simulink model "Controller_PP_testV1"  (R2021a)
settings: Solver=FixedStepDiscrete  StartTime=0.0  StopTime=inf  FixedStep=0.05  RelTol=1e-3
PostLoadFcn:
  | , if any(exist('dsrtsu_mdlpostloadfcn', 'file') == [2, 3, 6]), try dsrtsu_mdlpostloadfcn('Execute', bdroot); catch fprintf('Error in PostLoadFcn (dsrtsu_mdlpostloadfcn) for model "%s":\n %s\n', bdroot, lasterr); end, end,
model workspace (MAT data in the model file):
  DLC_kr = [-5.84862481044e-05 -6.43095507895e-05 -7.01328534794e-05 -7.5956156174e-05 -8.17794588731e-05 -8.76027615758e-05 -9.34260642811e-05 -9.92493669872e-05 -0.000105072669692 -0.000110895972393 -0.000116719275087 -0.000122542545808 ... (2080 elements, 1x2080)]
  DLC_thetar = [1.57172954906 1.57172588114 1.57172186534 1.57171750165 1.57171279008 1.57170773062 1.57170232328 1.57169656806 1.57169046495 1.57168401395 1.57167721507 1.57167006831 ... (2080 elements, 1x2080)]
  DLC_xr = [-0.00056695162723 -0.000622594591628 -0.000678008043004 -0.000733171198692 -0.000788063276025 -0.000842663492338 -0.000896951064963 -0.000950905211235 -0.00100450514849 -0.00105773009405 -0.00111055926527 -0.00116297187948 ... (2080 elements, 1x2080)]
  DLC_yr = [0.59999973213 0.659739817002 0.719479902091 0.779219987412 0.838960072984 0.898700158824 0.958440244948 1.01818033138 1.07792041812 1.1376605052 1.19740059264 1.25714068045 ... (2080 elements, 1x2080)]
  Fliter_ = 0.5
  Fliter_k = 1
  Iz = 1650
  SL_ROS_VariableLengthArrays_MaxSizes : object (value not decoded)
  a = 1
  b = 1.8
  cf = -120000
  cr = -120000
  factor_str = 0.15
  k1 = [0.258198889801 0.258198889749 0.258198889743 0.258198889805 0.258198889772 0.258198889764 0.258198889767 0.258198889768 0.258198889748 0.258198889747 0.258198889747 0.258198889747 ... (1000 elements, 1x1000)]
  k2 = [0.000225641086743 0.000451280556994 0.000676916794375 0.000902548182649 0.00112817310577 0.00135378994806 0.00157939709421 0.00180499292937 0.00203057583924 0.00225614421016 0.00248169642913 0.00270723088396 ... (1000 elements, 1x1000)]
  k3 = [1.8072435186 1.8072437178 1.80724404966 1.8072445143 1.80724511184 1.80724584231 1.80724670582 1.80724770248 1.80724883243 1.8072500958 1.80725149277 1.80725302351 ... (1000 elements, 1x1000)]
  k4 = [0.000229144738699 0.000458288056581 0.000687428532897 0.000916564747031 0.00114569527856 0.00137481870732 0.00160393361347 0.00183303857755 0.00206213218056 0.00229121300401 0.00252027963002 0.00274933064131 ... (1000 elements, 1x1000)]
  kr = [3.43040952456 5.20354947673 6.57526776383 5.89663744443 5.05963864905 4.19207203133 3.37422700169 2.64183787985 2.00068698258 1.44046440991 0.943931458435 0.491794250204 ... (89883 elements, 89883x1)]
  m = 1500
  straight_kr = [0 0 0 0 0 0 0 0 0 0 0 0 ... (10000 elements, 10000x1)]
  straight_thetar = [1.5708 1.5708 1.5708 1.5708 1.5708 1.5708 1.5708 1.5708 1.5708 1.5708 1.5708 1.5708 ... (10000 elements, 10000x1)]
  straight_xr = [0 0 0 0 0 0 0 0 0 0 0 0 ... (10000 elements, 10000x1)]
  straight_yr = [0.01 0.02 0.03 0.04 0.05 0.06 0.07 0.08 0.09 0.1 0.11 0.12 ... (10000 elements, 10000x1)]
  thetar = [0.0108871889919 0.137918447215 0.259619297152 0.371627288769 0.47112102891 0.556859678388 0.628810120477 0.687658443901 0.734398145371 0.77005371967 0.795522448239 0.811495552059 ... (89883 elements, 89883x1)]
  xr = [399944.786619 399944.805491 399944.823621 399944.841077 399944.857922 399944.874223 399944.890046 399944.905456 399944.920519 399944.935301 399944.949866 399944.964282 ... (89883 elements, 89883x1)]
  xr_init = 3407363.99438
  yr = [3406937.32043 3406937.32184 3406937.3255 3406937.33122 3406937.33879 3406937.34802 3406937.35871 3406937.37066 3406937.38366 3406937.39752 3406937.41203 3406937.427 ... (89883 elements, 89883x1)]
  yr_init = 400335.964759
undefined symbols (not defined in the file or in its folder): Data, Data_SL_Info
libraries: robotlib x5, simulink_extras x3
(part 2 of 2)

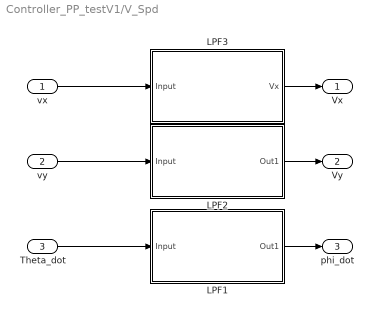
== system Controller_PP_testV1/V_Spd ==
  vx : Inport
  vy : Inport  Port=2
  Theta_dot : Inport  Port=3
  LPF1 : Subsystem  TreatAsAtomicUnit=on
  LPF2 : Subsystem  TreatAsAtomicUnit=on
  LPF3 : Subsystem  TreatAsAtomicUnit=on
  Vx : Outport  VectorParamsAs1DForOutWhenUnconnected=off
  Vy : Outport  Port=2  VectorParamsAs1DForOutWhenUnconnected=off
  phi_dot : Outport  Port=3  VectorParamsAs1DForOutWhenUnconnected=off
  wires:
  Theta_dot/1 -> LPF1/1(Input)
  LPF1/1(Out1) -> phi_dot/1
  LPF2/1(Out1) -> Vy/1
  LPF3/1(Vx) -> Vx/1
  vx/1 -> LPF3/1(Input)
  vy/1 -> LPF2/1(Input)

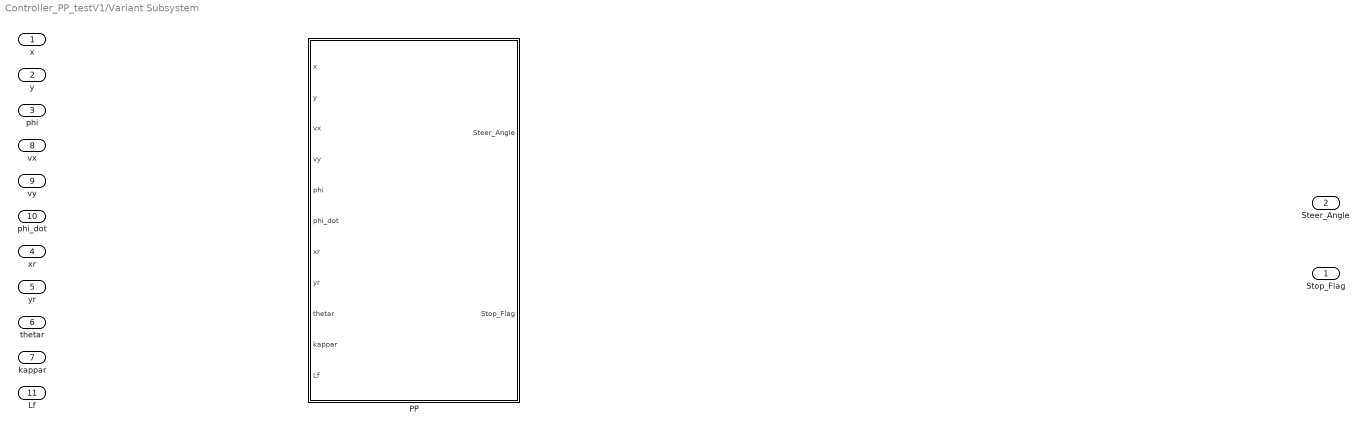
== system Controller_PP_testV1/Variant Subsystem ==
  x : Inport
  y : Inport  Port=2
  phi : Inport  Port=3
  xr : Inport  Port=4
  yr : Inport  Port=5
  thetar : Inport  Port=6
  kappar : Inport  Port=7
  vx : Inport  Port=8
  vy : Inport  Port=9
  phi_dot : Inport  Port=10
  Lf : Inport  Port=11
  PP : Subsystem  VariantControl=Controller == 5
  Stop_Flag : Outport  VectorParamsAs1DForOutWhenUnconnected=off
  Steer_Angle : Outport  Port=2  VectorParamsAs1DForOutWhenUnconnected=off

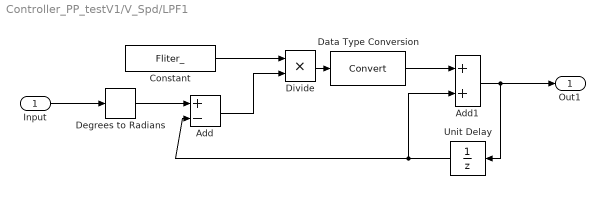
== system Controller_PP_testV1/V_Spd/LPF1 ==
  Input : Inport
  Add : Sum  Inputs=+-
  Add1 : Sum
  Constant : Constant  Value=Fliter_
  Data Type Conversion : DataTypeConversion
  Degrees to Radians : simulink_extras/Transformations/Degrees to Radians
  Divide : Product  Inputs=**
  Unit Delay : UnitDelay  SampleTime=-1  HasFrameUpgradeWarning=on
  Out1 : Outport  VectorParamsAs1DForOutWhenUnconnected=off
  wires:
  Divide/1 -> Data Type Conversion/1
  Input/1 -> Degrees to Radians/1
  Constant/1 -> Divide/1
  Add/1 -> Divide/2
  Data Type Conversion/1 -> Add1/1
  Add1/1 -> Unit Delay/1, Out1/1
  Unit Delay/1 -> Add/2, Add1/2
  Degrees to Radians/1 -> Add/1

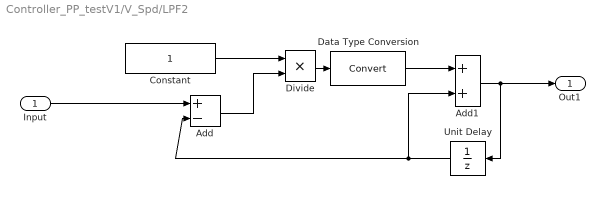
== system Controller_PP_testV1/V_Spd/LPF2 ==
  Input : Inport
  Add : Sum  Inputs=+-
  Add1 : Sum
  Constant : Constant
  Data Type Conversion : DataTypeConversion
  Divide : Product  Inputs=**
  Unit Delay : UnitDelay  SampleTime=-1  HasFrameUpgradeWarning=on
  Out1 : Outport  VectorParamsAs1DForOutWhenUnconnected=off
  wires:
  Divide/1 -> Data Type Conversion/1
  Constant/1 -> Divide/1
  Add/1 -> Divide/2
  Data Type Conversion/1 -> Add1/1
  Add1/1 -> Unit Delay/1, Out1/1
  Unit Delay/1 -> Add/2, Add1/2
  Input/1 -> Add/1

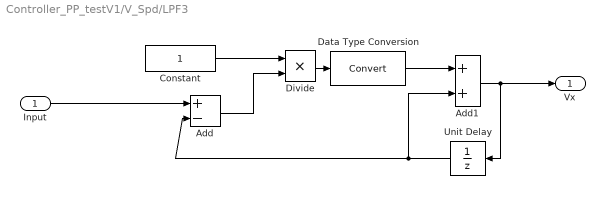
== system Controller_PP_testV1/V_Spd/LPF3 ==
  Input : Inport
  Add : Sum  Inputs=+-
  Add1 : Sum
  Constant : Constant
  Data Type Conversion : DataTypeConversion
  Divide : Product  Inputs=**
  Unit Delay : UnitDelay  SampleTime=-1  HasFrameUpgradeWarning=on
  Vx : Outport  VectorParamsAs1DForOutWhenUnconnected=off
  wires:
  Input/1 -> Add/1
  Unit Delay/1 -> Add1/2, Add/2
  Add1/1 -> Vx/1, Unit Delay/1
  Data Type Conversion/1 -> Add1/1
  Add/1 -> Divide/2
  Constant/1 -> Divide/1
  Divide/1 -> Data Type Conversion/1

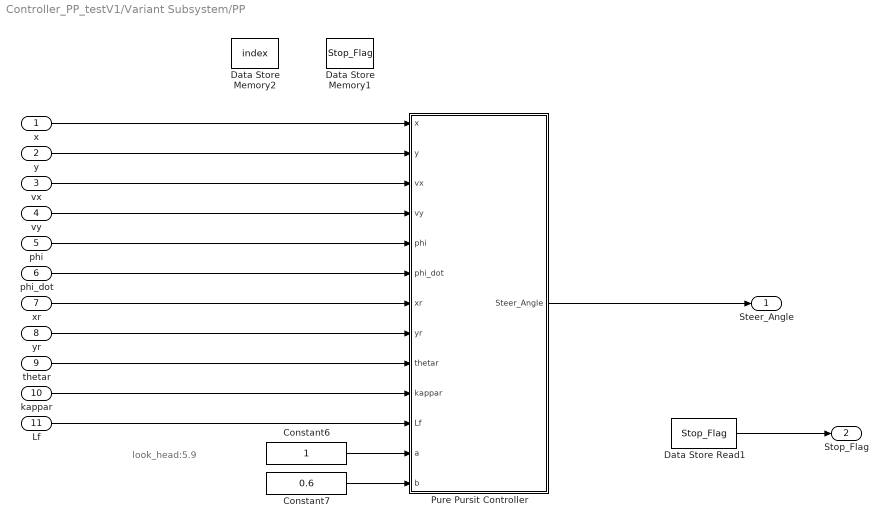
== system Controller_PP_testV1/Variant Subsystem/PP ==
  note: look_head:5.9
  x : Inport
  y : Inport  Port=2
  vx : Inport  Port=3
  vy : Inport  Port=4
  phi : Inport  Port=5
  phi_dot : Inport  Port=6
  xr : Inport  Port=7
  yr : Inport  Port=8
  thetar : Inport  Port=9
  kappar : Inport  Port=10
  Lf : Inport  Port=11
  Constant6 : Constant
  Constant7 : Constant  Value=0.6
  Data Store Memory1 : DataStoreMemory  DataStoreName=Stop_Flag  ReadBeforeWriteMsg=warning  WriteAfterWriteMsg=warning  WriteAfterReadMsg=warning  ShowAdditionalParam=off  OutDataTypeStr=double
  Data Store Memory2 : DataStoreMemory  DataStoreName=index  ReadBeforeWriteMsg=warning  WriteAfterWriteMsg=warning  WriteAfterReadMsg=warning  ShowAdditionalParam=off  OutDataTypeStr=double
  Data Store Read1 : DataStoreRead  DataStoreName=Stop_Flag  IndexOptions=Index vector (dialog)  Indices=1  OutputSizes=1
  Pure Pursit Controller : MATLAB Function  TreatAsAtomicUnit=on
  Steer_Angle : Outport
  Stop_Flag : Outport  Port=2
  wires:
  phi_dot/1 -> Pure Pursit Controller/6(phi_dot)
  Constant7/1 -> Pure Pursit Controller/13(b)
  vx/1 -> Pure Pursit Controller/3(vx)
  y/1 -> Pure Pursit Controller/2(y)
  thetar/1 -> Pure Pursit Controller/9(thetar)
  xr/1 -> Pure Pursit Controller/7(xr)
  Constant6/1 -> Pure Pursit Controller/12(a)
  vy/1 -> Pure Pursit Controller/4(vy)
  yr/1 -> Pure Pursit Controller/8(yr)
  x/1 -> Pure Pursit Controller/1(x)
  kappar/1 -> Pure Pursit Controller/10(kappar)
  Pure Pursit Controller/1(Steer_Angle) -> Steer_Angle/1
  phi/1 -> Pure Pursit Controller/5(phi)
  Data Store Read1/1 -> Stop_Flag/1
  Lf/1 -> Pure Pursit Controller/11(Lf)

== matlab function Controller_PP_testV1/MATLAB Function ==
  data: u input; xr output; yr output
function [xr,yr] = fcn(u)
xr = u(:,1);
yr = u(:,2);
end

== matlab function Controller_PP_testV1/MATLAB Function1 ==
  data: x input; y input; cones_real_heading input; cones_real_center_x input; cones_real_center_y input; new_pose data_store_memory

function fcn(x,y,cones_real_heading,cones_real_center_x,cones_real_center_y)
coder.extrinsic('plot');
%coder.extrinsic('equal');
star_pose_x = 0;   %先验8字绕环车辆起始x位置 m
star_pose_y = -2.5;%先验8字绕环车辆起始y位置 m
r = 9.125;         %先验8字绕环圆的半径
lane_width = 3;    %先验8字绕环车道宽 m
% cones_interval = 5;%先验8字绕环纵向锥桶间距 m
persistent flag  
if isempty(flag)
    flag = 0;
end
global new_pose
%% 建立先验8字路径
if flag == 0
    refPoses = zeros(191,2);
    cones_origin_poses = zeros(4,2);
    index =1;
    refPoses(1,:)=[star_pose_x,star_pose_y];
    for i =1:10
        refPoses(index+i,:)=[star_pose_x,star_pose_y+1.3*i];
    end
    index = index+20;
    for i=1:20
         refPoses(index+i,:)=[star_pose_x+r-r*cos(i*(pi/20)),r*sin(i*(pi/20))+15+star_pose_y];
    end
    index=index+20;
    for i=1:20
         refPoses(index+i,:)=[star_pose_x+r-r*cos(pi+i*(pi/20)),r*sin(pi+i*(pi/20))+15+star_pose_y];
    end
    index=index+20;
    for i=1:20
         refPoses(index+i,:)=[star_pose_x+r-r*cos(i*(pi/20)),r*sin(i*(pi/20))+15+star_pose_y];
    end
    index=index+20;
    for i=1:20
         refPoses(index+i,:)=[star_pose_x+r-r*cos(pi+i*(pi/20)),r*sin(pi+i*(pi/20))+15+star_pose_y];
    end
    index=index+20;
    for i=1:20
        refPoses(index+i,:)=[star_pose_x-r+r*cos(i*(pi/20)),r*sin(i*(pi/20))+15+star_pose_y];
    end
    index=index+20;
    for i=1:20
        refPoses(index+i,:)=[star_pose_x-r+r*cos(pi+i*(pi/20)),r*sin(pi+i*(pi/20))+15+star_pose_y];
    end
    index=index+20;
    for i=1:20
        refPoses(index+i,:)=[star_pose_x-r+r*cos(i*(pi/20)),r*sin(i*(pi/20))+15+star_pose_y];
    end
    index=index+20;
    for i=1:20
        refPoses(index+i,:)=[star_pose_x-r+r*cos(pi+i*(pi/20)),r*sin(pi+i*(pi/20))+15+star_pose_y];
    end
    index=index+20;
    for i =1:10
        refPoses(index+i,:)=[star_pose_x,star_pose_y+17+1.3*i];
    end
%     index =1;
%     refPoses(1,:)=[star_pose_x,star_pose_y];
%     for i =1:5
%         refPoses(index+i,:)=[star_pose_x,star_pose_y+2.6*i];
%     end
%     index = index+5;
%     for i=1:10
%          refPoses(index+i,:)=[star_pose_x+r-r*cos(i*(pi/10)),r*sin(i*(pi/10))+15+star_pose_y];
%     end
%     index=index+10;
%     for i=1:10
%          refPoses(index+i,:)=[star_pose_x+r-r*cos(pi+i*(pi/10)),r*sin(pi+i*(pi/10))+15+star_pose_y];
%     end
%     index=index+10;
%     for i=1:10
%          refPoses(index+i,:)=[star_pose_x+r-r*cos(i*(pi/10)),r*sin(i*(pi/10))+15+star_pose_y];
%     end
%     index=index+10;
%     for i=1:10
%          refPoses(index+i,:)=[star_pose_x+r-r*cos(pi+i*(pi/10)),r*sin(pi+i*(pi/10))+15+star_pose_y];
%     end
%     index=index+10;
%     for i=1:10
%         refPoses(index+i,:)=[star_pose_x-r+r*cos(i*(pi/10)),r*sin(i*(pi/10))+15+star_pose_y];
%     end
%     index=index+10;
%     for i=1:10
%         refPoses(index+i,:)=[star_pose_x-r+r*cos(pi+i*(pi/10)),r*sin(pi+i*(pi/10))+15+star_pose_y];
%     end
%     index=index+10;
%     for i =1:5
%         refPoses(index+i,:)=[star_pose_x,star_pose_y+17+2.6*i];
%     end
    %figure(1);
    %% 建立先验初始4个黄色锥桶位置
    cones_poses = [star_pose_x-lane_width/2,star_pose_y; %根据赛道初始位置确定4个锥桶位置。
                   star_pose_x+lane_width/2,star_pose_y;
                   star_pose_x-lane_width/2,star_pose_y+5;
                   star_pose_x+lane_width/2,star_pose_y+5;];
    
%    plot(cones_poses(:,1),cones_poses(:,2),'ro'); %画锥桶
 %   axis equal;
 %   hold on;
  %   plot(refPoses(:,1),refPoses(:,2),'bo');%画路径
    %% 建立假设实际4个黄色锥桶的位置
    %模拟4个锥桶位置，通过平移旋转先验锥桶位置，并且添加随机数模拟实际摆放误差。
    %先求出4个黄色锥桶的重心位置
    cones_center_origin_x =sum(cones_poses(:,1))/4;
    cones_center_origin_y =sum(cones_poses(:,2))/4;
%   plot(cones_center_origin_x,cones_center_origin_y,'*');
    %确定当前4个锥桶的方位角(航向角)
    cones_origin_heading = atan2d(refPoses(2,2) -refPoses(1,2) ,refPoses(2,1) -refPoses(1,1));
    diff_cones_heading =-(cones_real_heading - cones_origin_heading);
    %先将锥桶重心平移到原点
    cones_origin_poses(:,1) = cones_poses(:,1) - cones_center_origin_x;
    cones_origin_poses(:,2) = cones_poses (:,2)- cones_center_origin_y;
    %旋转
    eul = [deg2rad(diff_cones_heading) 0 0];
    rotation_matrix_ = eul2rotm(eul);
    rotation_matrix_ = rotation_matrix_(1:2,:);
    cones_poses_real = cones_origin_poses * rotation_matrix_;
    %从重心平移回先验锥桶重心
    cones_poses_real(:,1) = cones_poses_real(:,1) + cones_center_origin_x;
    cones_poses_real(:,2) = cones_poses_real(:,2) + cones_center_origin_y;
    %平移到期望预设锥桶位置
    cones_poses_real(:,1) = cones_poses_real(:,1) + (cones_real_center_x -cones_center_origin_x);
    cones_poses_real(:,2) = cones_poses_real(:,2) + (cones_real_center_y -cones_center_origin_y);
    %加上随机数，模拟锥桶摆放
    cones_poses_real(1,:) = cones_poses_real(1,:);
    cones_poses_real(2,:) = cones_poses_real(2,:);
    cones_poses_real(3,:) = cones_poses_real(3,:);
    cones_poses_real(4,:) = cones_poses_real(4,:);

    %画期望4个锥桶位置
    
%     plot(cones_poses_real(:,1),cones_poses_real(:,2),'o');
    %% 根据实际锥桶位置和先验锥桶位置得到旋转矩阵和平移矩阵
    new_pose = Skid(cones_poses,cones_poses_real,refPoses); %调用函数
    flag = 1;

end
plot(x,y,'k*');
hold on;
axis equal;
grid on;
plot(new_pose(:,1),new_pose(:,2),'ro'); %画现在的实际路径曲线
%% 支持CodeGen的函数，用于ROS C++ / Simulink
function New_refPoses = Skid(cones_pre_Pose,cones_real_Pose,refPoses)
%input:cones_pre/real_Pos 4by2 Matrix %4个锥桶的先验/实际位置
       %row1 first left cone;
       %row2 first right cone;
       %row3 second left cone;
       %row4 second right cone;
%input:refPoses:8字的先验路径
%output:New_refPoses: 8字的实际路径

New_refPoses = zeros(191,2);
pose_temp = zeros(191,2);
%1.根据4个实际锥桶位置计算实际4个锥桶的方位角,重心坐标
cones_real_mid_x_1 = (cones_real_Pose(1,1)+ cones_real_Pose(2,1))/2;
cones_real_mid_y_1 = (cones_real_Pose(1,2)+ cones_real_Pose(2,2))/2;
cones_real_mid_x_2 = (cones_real_Pose(3,1)+ cones_real_Pose(4,1))/2;
cones_real_mid_y_2 = (cones_real_Pose(3,2)+ cones_real_Pose(4,2))/2;
diff_cones_real_x = cones_real_mid_x_2 - cones_real_mid_x_1;
diff_cones_real_y = cones_real_mid_y_2 - cones_real_mid_y_1;
cones_real_heading = atan2d(diff_cones_real_y,diff_cones_real_x);
cones_real_center_x =sum(cones_real_Pose(:,1))/4;
cones_real_center_y =sum(cones_real_Pose(:,2))/4;
%2..根据4个先验锥桶位置计算实际4个锥桶的方位角，重心坐标
cones_pre_mid_x_1 = (cones_pre_Pose(1,1)+ cones_pre_Pose(2,1))/2;
cones_pre_mid_y_1 = (cones_pre_Pose(1,2)+ cones_pre_Pose(2,2))/2;
cones_pre_mid_x_2 = (cones_pre_Pose(3,1)+ cones_pre_Pose(4,1))/2;
cones_pre_mid_y_2 = (cones_pre_Pose(3,2)+ cones_pre_Pose(4,2))/2;
diff_cones_pre_x = cones_pre_mid_x_2 - cones_pre_mid_x_1;
diff_cones_pre_y = cones_pre_mid_y_2 - cones_pre_mid_y_1;
cones_pre_heading = atan2d(diff_cones_pre_y ,diff_cones_pre_x);
cones_pre_center_x = sum(cones_pre_Pose(:,1))/4;
cones_pre_center_y = sum(cones_pre_Pose(:,2))/4;
%3 .计算方位偏差并计算旋转矩阵
diff_heading = -(cones_real_heading - cones_pre_heading); %deg
eu1 = [deg2rad(diff_heading) 0 0];
rotmZYX = eul2rotm(eu1);
%4 .将参考路径所有点减去实际锥桶重心后再进行旋转
refPoses(:,1) = refPoses(:,1) - cones_pre_center_x;
refPoses(:,2) = refPoses(:,2) - cones_pre_center_y;
pose_temp(:,:) = refPoses * rotmZYX(1:2,1:2);
pose_temp(:,1) = pose_temp(:,1) + cones_pre_center_x;
pose_temp(:,2) = pose_temp(:,2) + cones_pre_center_y;
%平移到实际位置
diff_x = cones_real_center_x - cones_pre_center_x; %两重心位置之差
diff_y = cones_real_center_y - cones_pre_center_y; %两重心位置之差
pose_temp(:,1) = pose_temp(:,1) + diff_x;
pose_temp(:,2) = pose_temp(:,2) + diff_y;
New_refPoses(:,:) = pose_temp(:,:);
end
end

== matlab function Controller_PP_testV1/MATLAB Function2 ==
  data: u input; y output; left_factor input; right_factor input
function y = fcn(u,left_factor,right_factor)
if u>=110 && u<=130
    y = u;
elseif u>=130 && u<=240
    y = left_factor*u;
else
    y = right_factor*u;
    
end
end

== matlab function Controller_PP_testV1/Variant Subsystem/PP/Pure Pursit Controller ==
  settings: updateMethod=DISCRETE
  data: x input; Steer_Angle output; y input; vx input; vy input; phi input; phi_dot input; xr input; yr input; thetar input; kappar input; Lf input; a input; b input; index data_store_memory; Stop_Flag data_store_memory
function Steer_Angle = fcn(x,y,vx,vy,phi,phi_dot,xr,yr,thetar,kappar, Lf,a,b)
global index;
global Stop_Flag;
% dmin=1;
% d_min_last = 1;
% for i = 1:n
%     d_min = (x-xr(i))^2+(y-yr(i))^2;
%     if d_min < d_min_last
%         dmin = i;
%         d_min_last = d_min;
%     end
% end
n = length(xr);
min=1;
    if index == 0  %%Code has not run yet;
		d_min=(x-xr(1))^2+(y-yr(1))^2;
		min=1;
		for i=1:20 %% search 1-20 points when car is running.
			d=(x-xr(i))^2+(y-yr(i))^2;
			if d<d_min
				d_min=d;
				min=i;
			end
		end
		dmin=min;
		index = dmin; %% dmin assigns to index;
    else
		d_min = (x-xr(index))^2+(y-yr(index))^2;
		min = index;
		if index <= n - 20
          for i = index:index+20
            d=(x-xr(i))^2+(y-yr(i))^2;
                if d<d_min
                    d_min=d;
                    min=i;
                end
          end
			dmin=min;
			index = dmin; %% dmin assigns to index;
		else 
			for i = index:n
				d=(x-xr(i))^2+(y-yr(i))^2;
				if d<d_min
					d_min=d;
					min=i;
                    if min == n-5
                        Stop_Flag =1;
                    end
				end
			end
			dmin=min;
			index = dmin; %% dmin assigns to index;
		end
    end



%     tor=[cos(thetar(dmin));sin(thetar(dmin))];
%     nor=[-sin(thetar(dmin));cos(thetar(dmin))];
%     d_err=[x-xr(dmin);y-yr(dmin)];
%     ed=nor'*d_err;
%     es=tor'*d_err;
%     projection_point_thetar=thetar(dmin)+kappar(dmin)*es;
%     ed_dot=vy*cos(phi-projection_point_thetar)+vx*sin(phi-projection_point_thetar);
%     ephi=sin(phi-projection_point_thetar);
%     s_dot1=vx*cos(phi-projection_point_thetar)-vy*sin(phi-projection_point_thetar);
%     s_dot=s_dot1/(1-kappar(dmin)*ed);
%     ephi_dot=phi_dot-kappar(dmin)*s_dot;
%     kr=kappar(dmin);
%     err=[ed;ed_dot;ephi;ephi_dot]; 
    
    L = 0.0; %Look ahead distance
    index_now = index;
    while Lf > L && (index_now + 1) < n                %计算思想：找到与当前位置最近的那个全局路径参考点前方预设预瞄距离的点，返回其在全局路径上的矩阵索引位。确定预瞄点
        L=sqrt((x-xr(index_now))^2+(y-yr(index_now))^2);
       % L = norm(curpos(1,1:2)-repos(index,1:2));
        index_now =index_now+1;
        %disp("%d",ind)
    end

    xr_LD =xr(index_now);%确定要跟踪的预瞄点坐标
    yr_LD =yr(index_now);
    Lateral_Err = (a+b)*sin(atan2((yr_LD-y),(xr_LD-x))  - phi);
    Steer_Angle = atan(2*Lateral_Err/Lf);
end
